simulink model "Simulink_Converters_Model"  (R2020a)
settings: Solver=VariableStepAuto  StartTime=0.0  StopTime=0.02  RelTol=1e-3
libraries: powerlib x9
settings Model: Creator=Ricardo Romero  LastModifiedBy=Ricardo Romero

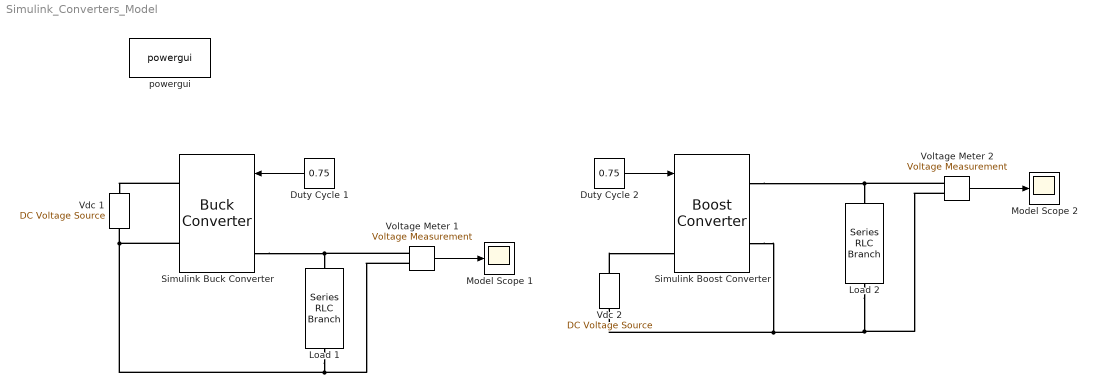
== system Simulink_Converters_Model ==
  Duty Cycle 1 : Constant  Value=0.75
  Duty Cycle 2 : Constant  Value=0.75
  Load 1 : powerlib/Elements/Series RLC Branch  LConnTagsString=__new0  RConnTagsString=__new0  BranchType=R  Resistance=10  Inductance=1e-3  SetiL0=off  InitialCurrent=0  Capacitance=1e-6  Setx0=off  InitialVoltage=0  Measurements=None
  Load 2 : powerlib/Elements/Series RLC Branch  LConnTagsString=__new0  RConnTagsString=__new0  BranchType=R  Resistance=10  Inductance=1e-3  SetiL0=off  InitialCurrent=0  Capacitance=1e-6  Setx0=off  InitialVoltage=0  Measurements=None
  Model Scope 1 : Scope
  Model Scope 2 : Scope
  Simulink Boost Converter : powerlib/Power Electronics/Boost Converter  ModelType=Average model (D-controlled)  Ron=1e-3  Rs=1e6  Cs=inf  Vforward=[0,0]  Ron_Diode=1e-3  Rs_Diode=1e6  Cs_Diode=inf  Vf_Diode=1e-3  Rs_CurrentSource=inf
      settings: SourceProductBaseCode=PS
  Simulink Buck Converter : powerlib/Power Electronics/Buck Converter  ModelType=Average model (D-controlled)  Ron=1e-3  Rs=1e6  Cs=inf  Vforward=[0,0]  Ron_Diode=1e-3  Rs_Diode=1e6  Cs_Diode=inf  Vf_Diode=1e-3  Rs_CurrentSource=inf
      settings: SourceProductBaseCode=PS
  Vdc 1 : powerlib/Electrical Sources/DC Voltage Source  Amplitude=100  Measurements=None
  Vdc 2 : powerlib/Electrical Sources/DC Voltage Source  Amplitude=100  Measurements=None
  Voltage Meter 1 : powerlib/Measurements/Voltage Measurement  PhasorSimulation=off  OutputType=Complex  PSBequivalent=0
  Voltage Meter 2 : powerlib/Measurements/Voltage Measurement  PhasorSimulation=off  OutputType=Complex  PSBequivalent=0
  powergui : powerlib/powergui  Priority=1  SimulationMode=Continuous  SampleTime=50e-6  frequency=60  Iterations=50  frequencyindice=0  Pbase=100e6  ErrMax=1e-4  UnitsV=kV  UnitsW=MW  buscounter=0  FunctionMessages=off  echomessages=off  EnableUseOfTLC=off  CurrentSourceSwitches=off  DisableSnubberDevices=off  DisableRonSwitches=off  DisableVfSwitches=off  DisplayEquations=off  AutomaticDiscreteSolvers=off  SolverType=Tustin/Backward Euler (TBE)  Interpol=off  ExternalGateDelay=off  methode=off  Ts=100  x0status=blocks  SPID=on  SwTol=0  HookPort=off  NonlinearTolerance=1e-4  nMaxIteration=100  ContinueOnMaxIteration=off  RestoreLinks=warning  ResistiveCurrentMeasurement=off  Frange=[0:2:500]  Ylog=off  Xlog=on  ShowGrid=off  save=off  variable=ZData  structure=0  ZoomFFT=off  StartTime=0.0  cycles=1  DisplayStyle=1  fundamental=60  FreqAxis=off  MaxFrequency=1000  frequencyindicesteady=1  RmsSteady=1  display=off
  wires:
  Duty Cycle 1/1 -> Simulink Buck Converter/1
  Voltage Meter 1/1 -> Model Scope 1/1
  Duty Cycle 2/1 -> Simulink Boost Converter/1
  Voltage Meter 2/1 -> Model Scope 2/1
  connections:
  Simulink Buck Converter/RConn1 -- Vdc 1/RConn1
  Simulink Buck Converter/RConn2 -- Voltage Meter 1/LConn2 -- Load 1/RConn1 -- Vdc 1/LConn1
  Simulink Buck Converter/LConn1 -- Voltage Meter 1/LConn1 -- Load 1/LConn1
  Vdc 2/RConn1 -- Simulink Boost Converter/LConn1
  Simulink Boost Converter/RConn2 -- Voltage Meter 2/LConn2 -- Load 2/RConn1 -- Vdc 2/LConn1
  Simulink Boost Converter/RConn1 -- Load 2/LConn1 -- Voltage Meter 2/LConn1
